simulink model "TST_LIB_DYN_DRG"  (Simulink 8.8)
settings: Solver=VariableStepAuto  StartTime=0.0  StopTime=10.0  RelTol=1e-3
values from neighbouring files (symbols this model uses):
  atmdensity = 1.5e-12    [runTST_LIB_DYN_DRG.m]
  SCcom_MEC = [0; 0 ; 0]    [runTST_LIB_DYN_DRG.m]
undefined symbols (not defined in the file or in its folder): ATMvel_relBOF_BOF
libraries: LIB_DYN x1
settings Model: Creator=alger  LastModifiedBy=alger
settings DataIOCC: LimitDataPoints=off  SaveFormat=Dataset  SignalLoggingSaveFormat=Dataset
settings OptimizationCC: LifeSpan=auto
settings DebuggingCC: UnderspecifiedInitializationDetection=Simplified  MergeDetectMultiDrivingBlocksExec=error  FcnCallInpInsideContextMsg=error  StateNameClashWarn=none  SFUnexpectedBacktrackingDiag=error  SFNoUnconditionalDefaultTransitionDiag=error  SFExecutionAtInitializationDiag=warning
settings HardwareCC: ProdBitPerPointer=64  ProdBitPerSizeT=64  ProdBitPerPtrDiffT=64  ProdLargestAtomicFloat=Float  ProdIntDivRoundTo=Zero  ProdEndianess=LittleEndian  ProdWordSize=64  ProdHWDeviceType=Intel->x86-64 (Windows64)
settings ModelReferenceCC: PropagateSignalLabelsOutOfModel=on
settings GRTTargetCC: TargetLangStandard=C99 (ISO)  GeneratePreprocessorConditionals=Use local settings  CombineOutputUpdateFcns=on  GRTInterface=off
settings ConfigComp: CovMetricSettings=dwe  CovHtmlReporting=off  CovSaveCumulativeToWorkspaceVar=off  CovSaveSingleToWorkspaceVar=off  CovExternalEMLEnable=on

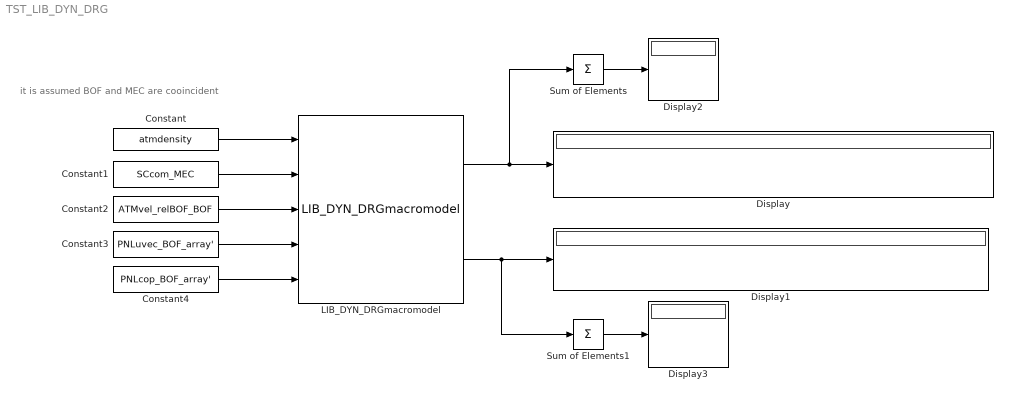
== system TST_LIB_DYN_DRG ==
  note: it is assumed BOF and MEC are cooincident
  Constant : Constant  Value=atmdensity
  Constant1 : Constant  Value=SCcom_MEC
  Constant2 : Constant  Value=ATMvel_relBOF_BOF
  Constant3 : Constant  Value=PNLuvec_BOF_array'
  Constant4 : Constant  Value=PNLcop_BOF_array'
  Display{,1..3} (4 alike) : Display
  "LIB_DYN_DRGmacromodel " : LIB_DYN/LIB_DYN_DRGmacromodel   N=6  pnlarea_array=PNLarea_array  pnlcd_array=PNLcd_array
  Sum of Elements : Sum  Inputs=+  CollapseMode=Specified dimension  CollapseDim=2
  Sum of Elements1 : Sum  Inputs=+  CollapseMode=Specified dimension  CollapseDim=2
  wires:
  Constant/1 -> "LIB_DYN_DRGmacromodel "/1
  Constant1/1 -> "LIB_DYN_DRGmacromodel "/2
  Constant2/1 -> "LIB_DYN_DRGmacromodel "/3
  Constant3/1 -> "LIB_DYN_DRGmacromodel "/4
  Constant4/1 -> "LIB_DYN_DRGmacromodel "/5
  "LIB_DYN_DRGmacromodel "/1 -> Sum of Elements/1, Display/1
  "LIB_DYN_DRGmacromodel "/2 -> Sum of Elements1/1, Display1/1
  Sum of Elements/1 -> Display2/1
  Sum of Elements1/1 -> Display3/1
